simulink model "MIMOController_Observer"  (R2015b)
settings: Solver=VariableStepAuto  StartTime=0.0  StopTime=Simulation_Time  RelTol=1e-3
values from neighbouring files (symbols this model uses):
  A = [0 1 0 0; 0 24.4 0 0; 0 0 0 1; 0 0 0 0]    [LinABCD.m]
  B = [0 0;12648.1 0; 0 0;-2011.69 -.444031]    [LinABCD.m]
  C = [1 0 0 0;0 0 1 0]    [LinABCD.m]
  K_bar1 = [K_bar(:,1:4)]    [LinABCD.m]
  K_bar2 = [-K_bar(:,5:6)]    [LinABCD.m]
  L = place(A',C',[-.1;-.4;-.1;-.5])'    [LinABCD.m]
  Simulation_step = 1    [LinABCD.m]
settings Model: Creator=dmartin_a  LastModifiedBy=dmartin_a

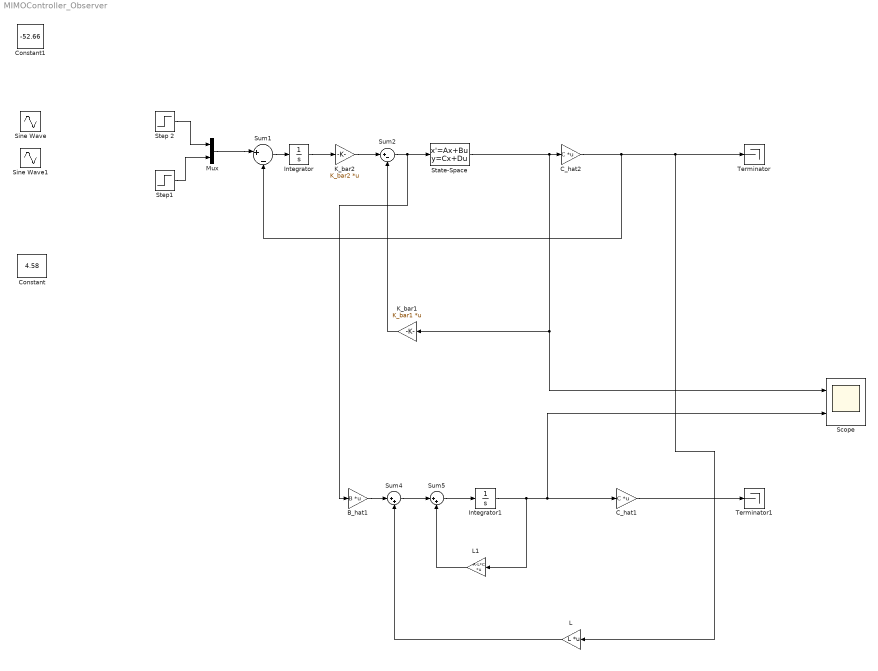
== system MIMOController_Observer ==
  B_hat1 : Gain  Gain=B  Multiplication=Matrix(K*u)
  C_hat1 : Gain  Gain=C  Multiplication=Matrix(K*u)
  C_hat2 : Gain  Gain=C  Multiplication=Matrix(K*u)
  Constant : Constant  Value=4.58
  Constant1 : Constant  Value=-52.66
  Integrator : Integrator  InitialCondition=[0 0]
  Integrator1 : Integrator  InitialCondition=[0 0 0 0]
  K_bar1 : Gain  Gain=K_bar1  Multiplication=Matrix(K*u)
  K_bar2 : Gain  Gain=K_bar2  Multiplication=Matrix(K*u)
  L : Gain  Gain=L  Multiplication=Matrix(K*u)
  L1 : Gain  Gain=A-L*C  Multiplication=Matrix(K*u)
  Mux : Mux  Inputs=2
  Scope : Scope  NumInputPorts=2
  Sine Wave : Sin  SampleTime=0
  Sine Wave1 : Sin  SampleTime=0
  State-Space : StateSpace  A=A  B=B  C=[1 0 0 0; 0 1 0 0; 0 0 1 0;0 0 0 1]  D=[0 0;0 0;0 0;0 0]  X0=[10 10 10 10]
  Step 2 : Step  Time=10  Before=5  After=10  SampleTime=Simulation_step
  Step1 : Step  Time=10  Before=6  After=11  SampleTime=Simulation_step
  Sum1 : Sum  Inputs=||+||-
  Sum2 : Sum  Inputs=|+-
  Sum4 : Sum  Inputs=|++
  Sum5 : Sum  Inputs=|++
  Terminator : Terminator
  Terminator1 : Terminator
  wires:
  K_bar1/1 -> Sum2/2
  Sum2/1 -> B_hat1/1, State-Space/1
  Step 2/1 -> Mux/1
  Step1/1 -> Mux/2
  L/1 -> Sum4/2
  Mux/1 -> Sum1/1
  Sum5/1 -> Integrator1/1
  Integrator1/1 -> L1/1, Scope/2, C_hat1/1
  L1/1 -> Sum5/2
  Sum4/1 -> Sum5/1
  B_hat1/1 -> Sum4/1
  State-Space/1 -> Scope/1, K_bar1/1, C_hat2/1
  Integrator/1 -> K_bar2/1
  Sum1/1 -> Integrator/1
  K_bar2/1 -> Sum2/1
  C_hat2/1 -> Sum1/2, L/1, Terminator/1
  C_hat1/1 -> Terminator1/1
